simulink model "Ellipse_Trajectory_Generator"  (R2023a)
settings: Solver=ode4  StartTime=0.0  StopTime=Tend  FixedStep=Ts  RelTol=1e-3
values from neighbouring files (symbols this model uses):
  a1 = 5    [trajectory_csv_generator.m]
  a2 = 3    [trajectory_csv_generator.m]
settings Model: Creator=PhDstudent1  LastModifiedBy=Juan Augusto Paredes
settings ModelReferenceCC: EnableRefExpFcnMdlSchedulingChecks=on

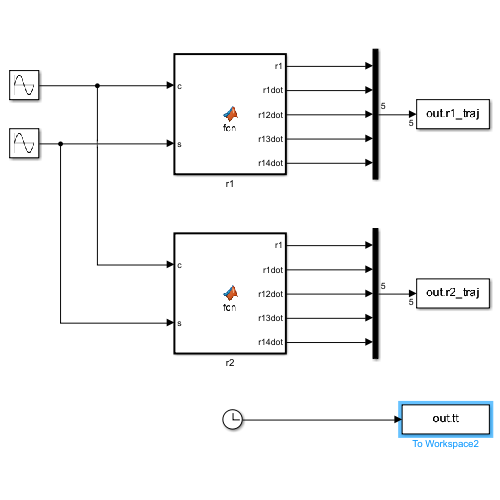
[thumbnail: Simulink's stored preview of the top-level diagram]
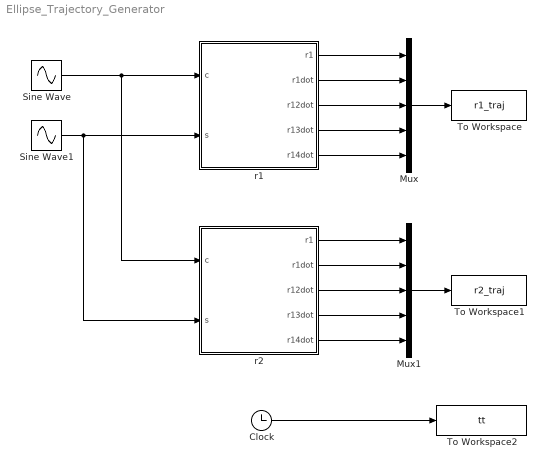
== system Ellipse_Trajectory_Generator ==
  Clock : Clock
  Mux : Mux  Inputs=5
  Mux1 : Mux  Inputs=5
  Sine Wave : Sin  Phase=pi/2  SampleTime=0
  Sine Wave1 : Sin  SampleTime=0
  To Workspace : ToWorkspace  VariableName=r1_traj  SampleTime=-1
  To Workspace1 : ToWorkspace  VariableName=r2_traj  SampleTime=-1
  To Workspace2 : ToWorkspace  VariableName=tt  SampleTime=-1
  r1 : MATLAB Function  TreatAsAtomicUnit=on
  r2 : MATLAB Function  TreatAsAtomicUnit=on
  wires:
  r2/5(r14dot) -> Mux1/5
  r2/4(r13dot) -> Mux1/4
  r2/3(r12dot) -> Mux1/3
  r2/2(r1dot) -> Mux1/2
  r2/1(r1) -> Mux1/1
  r1/5(r14dot) -> Mux/5
  r1/4(r13dot) -> Mux/4
  r1/3(r12dot) -> Mux/3
  r1/2(r1dot) -> Mux/2
  r1/1(r1) -> Mux/1
  Sine Wave1/1 -> r2/2(s), r1/2(s)
  Sine Wave/1 -> r2/1(c), r1/1(c)
  Mux/1 -> To Workspace/1
  Mux1/1 -> To Workspace1/1
  Clock/1 -> To Workspace2/1

== matlab function Ellipse_Trajectory_Generator/r1 ==
  data: c input size=1; r1 output size=1; s input size=1; r1dot output size=1; r12dot output size=1; r13dot output size=1; r14dot output size=1; a2 parameter size=1; a1 parameter size=1
function [r1,r1dot,r12dot,r13dot,r14dot] = fcn(c,s,a2, a1)

%a1 = 5;
%a2 = 3;

r1 = a1*sqrt(2)/2 - a1*sqrt(2)*c/2 - a2*sqrt(2)*s/2;
r1dot = a1*sqrt(2)*s/2 - a2*sqrt(2)*c/2;
r12dot = a1*sqrt(2)*c/2 + a2*sqrt(2)*s/2;
r13dot = -a1*sqrt(2)*s/2 + a2*sqrt(2)*c/2;
r14dot = -a1*sqrt(2)*c/2 - a2*sqrt(2)*s/2;
end

== matlab function Ellipse_Trajectory_Generator/r2 ==
  data: c input size=1; r1 output size=1; s input size=1; r1dot output size=1; r12dot output size=1; r13dot output size=1; r14dot output size=1; a1 parameter size=1; a2 parameter size=1
function [r1,r1dot,r12dot,r13dot,r14dot] = fcn(c,s,a1, a2)

%a1 = 5;
%a2 = 3;

r1 = a1*sqrt(2)/2 - a1*sqrt(2)*c/2 + a2*sqrt(2)*s/2;
r1dot = a1*sqrt(2)*s/2 + a2*sqrt(2)*c/2;
r12dot = a1*sqrt(2)*c/2 - a2*sqrt(2)*s/2;
r13dot = -a1*sqrt(2)*s/2 - a2*sqrt(2)*c/2;
r14dot = -a1*sqrt(2)*c/2 + a2*sqrt(2)*s/2;
end
